simulink model "IEEE123_4subsystem"  (R2022b)
settings: Solver=ode4  StartTime=0.0  StopTime=inf  FixedStep=Ts  MaxStep=1e-4  RelTol=1e-3
PreLoadFcn:
  | Ts = 50e-6;
PostLoadFcn:
  | Ts = 50e-6;
InitFcn:
  | %%%%%%%%%%%%%%%%%%%%%%%%
  | % Simulation data for the IEEE 123 Node Test Feeder model
  | %%%%%%%%%%%%%%%%%%%%%%%
  | 
  | % miles/km
  | mi2km = 1.60934;
  | 
  | % feet to km
  | ft2km = 0.0003048;
  | 
  | % microsiemens to Farads
  | ms2F = 1/2/pi/60*1e-6;
  | 
  | %% Configuration 1 - series reactance - ohm/mile
  | 
  | R_1 = [0.4576 0.1560 0.1535;0.1560 0.4666 0.1580;0.1535 0.1580 0.4615];
  | X_1 = [1.0780 0.5017 0.3849;0.5017 1.0482 0.4236;0.3849 0.4236 1.0651];
  | 
  | % charging susceptance - microsiemens/mile
  | 
  | B_1 = [5.6765 -1.8319 -0.6982;-1.8319 5.9809 -1.1645;-0.6982 -1.1645 5.3971];
  | 
  | % convert for SPS
  | 
  | R_1 = R_1/mi2km;
  | 
  | Rs_1=(R_1(1,1)+R_1(2,2)+R_1(3,3))/3;
  | Rm_1=(R_1(1,2)+R_1(1,3)+R_1(2,3))/3;
  | R1_1=Rs_1-Rm_1;
  | R0_1=Rs_1+2*Rm_1;
  | 
  | L_1 = X_1/mi2km/2/pi/60;
  | 
  | Ls_1=(L_1(1,1)+L_1(2,2)+L_1(3,3))/3;
  | Lm_1=(L_1(1,2)+L_1(1,3)+L_1(2,3))/3;
  | L1_1=Ls_1-Lm_1;
  | L0_1=Ls_1+2*Lm_1;
  | 
  | C_1 = B_1/mi2km*ms2F;
  | 
  | Cs_1=(C_1(1,1)+C_1(2,2)+C_1(3,3))/3;
  | Cm_1=(C_1(1,2)+C_1(1,3)+C_1(2,3))/3;
  | C1_1=Cs_1-Cm_1;
  | C0_1=Cs_1+2*Cm_1;
  | 
  | 
  | %% Configuration 2 - series reactance - ohm/mile
  | 
  | R_2 = [0.4666 0.1580 0.1560;0.1580 0.4615 0.1535;0.1560 0.1535 0.4576];
  | X_2 = [1.0482 0.4236 0.5017;0.4236 1.0651 0.3849;0.5017 0.3849 1.0780];
  | 
  | % charging susceptance - microsiemens/mile
  | 
  | B_2 = [5.9809 -1.1645 -1.8319;-1.1645 5.3971 -0.6982;-1.8319 -0.6982 5.6765];
  | 
  | % convert for SPS
  | 
  | R_2 = R_2/mi2km;
  | 
  | Rs_2=(R_2(1,1)+R_2(2,2)+R_2(3,3))/3;
  | Rm_2=(R_2(1,2)+R_2(1,3)+R_2(2,3))/3;
  | R1_2=Rs_2-Rm_2;
  | R0_2=Rs_2+2*Rm_2;
  | 
  | L_2 = X_2/mi2km/2/pi/60;
  | 
  | Ls_2=(L_2(1,1)+L_2(2,2)+L_2(3,3))/3;
  | Lm_2=(L_2(1,2)+L_2(1,3)+L_2(2,3))/3;
  | L1_2=Ls_2-Lm_2;
  | L0_2=Ls_2+2*Lm_2;
  | 
  | C_2 = B_2/mi2km*ms2F;
  | 
  | Cs_2=(C_2(1,1)+C_2(2,2)+C_2(3,3))/3;
  | Cm_2=(C_2(1,2)+C_2(1,3)+C_2(2,3))/3;
  | C1_2=Cs_2-Cm_2;
  | C0_2=Cs_2+2*Cm_2;
  | 
  | 
  | %% Configuration 3 - series reactance - ohm/mile
  | 
  | R_3 = [0.4615 0.1535 0.1580;0.1535 0.4576 0.1560;0.1580 0.1560 0.4666];
  | X_3 = [1.0651 0.3849 0.4236;0.3849 1.0780 0.5017;0.4236 0.5017 1.0482];
  | 
  | % charging susceptance - microsiemens/mile
  | 
  | B_3 = [5.3971 -0.6982 -1.1645;-0.6982 5.6765 -1.8319; -1.1645 -1.8319 5.9809];
  | 
  | % convert for SPS
  | 
  | R_3 = R_3/mi2km;
  | 
  | Rs_3=(R_3(1,1)+R_3(2,2)+R_3(3,3))/3;
  | Rm_3=(R_3(1,2)+R_3(1,3)+R_3(2,3))/3;
  | R1_3=Rs_3-Rm_3;
  | R0_3=Rs_3+2*Rm_3;
  | 
  | L_3 = X_3/mi2km/2/pi/60;
  | 
  | Ls_3=(L_3(1,1)+L_3(2,2)+L_3(3,3))/3;
  | Lm_3=(L_3(1,2)+L_3(1,3)+L_3(2,3))/3;
  | L1_3=Ls_3-Lm_3;
  | L0_3=Ls_3+2*Lm_3;
  | 
  | C_3 = B_3/mi2km*ms2F;
  | 
  | Cs_3=(C_3(1,1)+C_3(2,2)+C_3(3,3))/3;
  | Cm_3=(C_3(1,2)+C_3(1,3)+C_3(2,3))/3;
  | C1_3=Cs_3-Cm_3;
  | C0_3=Cs_3+2*Cm_3;
  | 
  | %% Configuration 4 - series reactance - ohm/mile
  | 
  | R_4 = [0.4615 0.1580 0.1535;0.1580 0.4666 0.1560;0.1535 0.1560 0.4576];
  | X_4 = [1.0651 0.4236 0.3849;0.4236 1.0482 0.5017;0.3849 0.5017 1.0780];
  | 
  | % charging susceptance - microsiemens/mile
  | 
  | B_4 = [5.3971 -1.1645 -0.6982;-1.1645 5.9809 -1.8319;-0.6982 -1.8319 5.6765];
  | 
  | % convert for SPS
  | 
  | R_4 = R_4/mi2km;
  | 
  | Rs_4=(R_4(1,1)+R_4(2,2)+R_4(3,3))/3;
  | Rm_4=(R_4(1,2)+R_4(1,3)+R_4(2,3))/3;
  | R1_4=Rs_4-Rm_4;
  | R0_4=Rs_4+2*Rm_4;
  | 
  | L_4 = X_4/mi2km/2/pi/60;
  | 
  | Ls_4=(L_4(1,1)+L_4(2,2)+L_4(3,3))/3;
  | Lm_4=(L_4(1,2)+L_4(1,3)+L_4(2,3))/3;
  | L1_4=Ls_4-Lm_4;
  | L0_4=Ls_4+2*Lm_4;
  | 
  | C_4 = B_4/mi2km*ms2F;
  | 
  | Cs_4=(C_4(1,1)+C_4(2,2)+C_4(3,3))/3;
  | Cm_4=(C_4(1,2)+C_4(1,3)+C_4(2,3))/3;
  | C1_4=Cs_4-Cm_4;
  | C0_4=Cs_4+2*Cm_4;
  | 
  | 
  | %% Configuration 5 - series reactance - ohm/mile
  | 
  | R_5 = [0.4666 0.1560 0.1580;0.1560 0.4576 0.1535;0.1580 0.1535 0.4615];
  | X_5 = [1.0482 0.5017 0.4236;0.5017 1.0780 0.3849;0.4236 0.3849 1.0651];
  | 
  | % charging susceptance - microsiemens/mile
  | 
  | B_5 = [5.9809 -1.8319 -1.1645;-1.8319 5.6765 -0.6982;-1.1645 -0.6982 5.3971];
  | 
  | % convert for SPS
  | 
  | R_5 = R_5/mi2km;
  | 
  | Rs_5=(R_5(1,1)+R_5(2,2)+R_5(3,3))/3;
  | Rm_5=(R_5(1,2)+R_5(1,3)+R_5(2,3))/3;
  | R1_5=Rs_5-Rm_5;
  | R0_5=Rs_5+2*Rm_5;
  | 
  | L_5 = X_5/mi2km/2/pi/60;
  | 
  | Ls_5=(L_5(1,1)+L_5(2,2)+L_5(3,3))/3;
  | Lm_5=(L_5(1,2)+L_5(1,3)+L_5(2,3))/3;
  | L1_5=Ls_5-Lm_5;
  | L0_5=Ls_5+2*Lm_5;
  | 
  | C_5 = B_5/mi2km*ms2F;
  | 
  | Cs_5=(C_5(1,1)+C_5(2,2)+C_5(3,3))/3;
  | Cm_5=(C_5(1,2)+C_5(1,3)+C_5(2,3))/3;
  | C1_5=Cs_5-Cm_5;
  | C0_5=Cs_5+2*Cm_5;
  | 
  | %% Configuration 6 - series reactance - ohm/mile
  | 
  | R_6 = [0.4576 0.1535 0.1560;0.1535 0.4615 0.1580;0.1560 0.1580 0.4666];
  | X_6 = [1.0780 0.3849 0.5017;0.3849 1.0651 0.4236;0.5017 0.4236 1.0482];
  | 
  | % charging susceptance - microsiemens/mile
  | 
  | B_6 = [5.6765 -0.6982 -1.8319;-0.6982 5.3971 -1.1645;-1.8319 -1.1645 5.9809];
  | 
  | % convert for SPS
  | 
  | R_6 = R_6/mi2km;
  | 
  | Rs_6=(R_6(1,1)+R_6(2,2)+R_6(3,3))/3;
  | Rm_6=(R_6(1,2)+R_6(1,3)+R_6(2,3))/3;
  | R1_6=Rs_6-Rm_6;
  | R0_6=Rs_6+2*Rm_6;
  | 
  | L_6 = X_6/mi2km/2/pi/60;
  | 
  | Ls_6=(L_6(1,1)+L_6(2,2)+L_6(3,3))/3;
  | Lm_6=(L_6(1,2)+L_6(1,3)+L_6(2,3))/3;
  | L1_6=Ls_6-Lm_6;
  | L0_6=Ls_6+2*Lm_6;
  | 
  | C_6 = B_6/mi2km*ms2F;
  | 
  | Cs_6=(C_6(1,1)+C_6(2,2)+C_6(3,3))/3;
  | Cm_6=(C_6(1,2)+C_6(1,3)+C_6(2,3))/3;
  | C1_6=Cs_6-Cm_6;
  | C0_6=Cs_6+2*Cm_6;
  | 
  | 
  | %% Configuration 7 - series reactance - ohm/mile
  | 
  | R_7 = [0.4576 0.0000 0.1535;0.0000 0.0000 0.0000;0.1535 0.0000 0.4615];
  | X_7 = [1.0780 0.0000 0.3849;0.0000 0.0000 0.0000;0.3849 0.0000 1.0651];
  | 
  | % charging susceptance - microsiemens/mile
  | 
  | B_7 = [5.1154 0.0000 -1.0549;0.0000 0.0000 0.0000;-1.0549 0.0000 5.1704];
  | 
  | % convert for SPS
  | 
  | R_7 = R_7/mi2km;
  | 
  | Rs_7=(R_7(1,1)+R_7(2,2)+R_7(3,3))/3;
  | Rm_7=(R_7(1,2)+R_7(1,3)+R_7(2,3))/3;
  | R1_7=Rs_7-Rm_7;
  | R0_7=Rs_7+2*Rm_7;
  | 
  | L_7 = X_7/mi2km/2/pi/60;
  | 
  | Ls_7=(L_7(1,1)+L_7(2,2)+L_7(3,3))/3;
  | Lm_7=(L_7(1,2)+L_7(1,3)+L_7(2,3))/3;
  | L1_7=Ls_7-Lm_7;
  | L0_7=Ls_7+2*Lm_7;
  | 
  | C_7 = B_7/mi2km*ms2F;
  | 
  | Cs_7=(C_7(1,1)+C_7(2,2)+C_7(3,3))/3;
  | Cm_7=(C_7(1,2)+C_7(1,3)+C_7(2,3))/3;
  | C1_7=Cs_7-Cm_7;
  | C0_7=Cs_7+2*Cm_7;
  | 
  | 
  | %% Configuration 8 - series reactance - ohm/mile
  | 
  | R_8 = [0.4576 0.1535 0.0000;0.1535 0.4615 0.0000;0.0000 0.0000 0.0000];
  | X_8 = [1.0780 0.3849 0.0000;0.3849 1.0651 0.0000;0.0000 0.0000 0.0000];
  | 
  | % charging susceptance - microsiemens/mile
  | 
  | B_8 = [5.1154 -1.0549 0.0000;-1.0549 5.1704 0.0000;0.0000 0.0000 0.0000];
  | 
  | % convert for SPS
  | 
  | R_8 = R_8/mi2km;
  | 
  | Rs_8=(R_8(1,1)+R_8(2,2)+R_8(3,3))/3;
  | Rm_8=(R_8(1,2)+R_8(1,3)+R_8(2,3))/3;
  | R1_8=Rs_8-Rm_8;
  | R0_8=Rs_8+2*Rm_8;
  | 
  | L_8 = X_8/mi2km/2/pi/60;
  | 
  | Ls_8=(L_8(1,1)+L_8(2,2)+L_8(3,3))/3;
  | Lm_8=(L_8(1,2)+L_8(1,3)+L_8(2,3))/3;
  | L1_8=Ls_8-Lm_8;
  | L0_8=Ls_8+2*Lm_8;
  | 
  | C_8 = B_8/mi2km*ms2F;
  | 
  | Cs_8=(C_8(1,1)+C_8(2,2)+C_8(3,3))/3;
  | Cm_8=(C_8(1,2)+C_8(1,3)+C_8(2,3))/3;
  | C1_8=Cs_8-Cm_8;
  | C0_8=Cs_8+2*Cm_8;
  | 
  | %% Configuration 9 - series reactance - ohm/mile
  | 
  | R_9 = [1.3292 0 0;0 0 0;0 0 0];
  | X_9 = [1.3475 0 0;0 0 0;0 0 0];
  | 
  | % charging susceptance - microsiemens/mile
  | 
  | B_9 = [4.5193 0 0;0 0 0;0 0 0];
  | 
  | % convert for SPS
  | 
  | R_9 = R_9/mi2km;
  | 
  | Rs_9=(R_9(1,1)+R_9(2,2)+R_9(3,3))/3;
  | Rm_9=(R_9(1,2)+R_9(1,3)+R_9(2,3))/3;
  | R1_9=Rs_9-Rm_9;
  | R0_9=Rs_9+2*Rm_9;
  | 
  | L_9 = X_9/mi2km/2/pi/60;
  | 
  | Ls_9=(L_9(1,1)+L_9(2,2)+L_9(3,3))/3;
  | Lm_9=(L_9(1,2)+L_9(1,3)+L_9(2,3))/3;
  | L1_9=Ls_9-Lm_9;
  | L0_9=Ls_9+2*Lm_9;
  | 
  | C_9 = B_9/mi2km*ms2F;
  | 
  | Cs_9=(C_9(1,1)+C_9(2,2)+C_9(3,3))/3;
  | Cm_9=(C_9(1,2)+C_9(1,3)+C_9(2,3))/3;
  | C1_9=Cs_9-Cm_9;
  | C0_9=Cs_9+2*Cm_9;
  | 
  | %% Configuration 10- series reactance - ohm/mile
  | 
  | R_10 = [0 0 0;0 1.3292 0;0 0 0];
  | X_10 = [0 0 0;0 1.3475 0;0 0 0];
  | 
  | % charging susceptance - microsiemens/mile
  | B_10 = [0 0 0;0 4.5193 0;0 0 0];
  | 
  | % convert for SPS
  | 
  | R_10 = R_10/mi2km;
  | 
  | Rs_10=(R_10(1,1)+R_10(2,2)+R_10(3,3))/3;
  | Rm_10=(R_10(1,2)+R_10(1,3)+R_10(2,3))/3;
  | R1_10=Rs_10-Rm_10;
  | R0_10=Rs_10+2*Rm_10;
  | 
  | L_10 = X_10/mi2km/2/pi/60;
  | 
  | Ls_10=(L_10(1,1)+L_10(2,2)+L_10(3,3))/3;
  | Lm_10=(L_10(1,2)+L_10(1,3)+L_10(2,3))/3;
  | L1_10=Ls_10-Lm_10;
  | L0_10=Ls_10+2*Lm_10;
  | 
  | C_10 = B_10/mi2km*ms2F;
  | 
  | Cs_10=(C_10(1,1)+C_10(2,2)+C_10(3,3))/3;
  | Cm_10=(C_10(1,2)+C_10(1,3)+C_10(2,3))/3;
  | C1_10=Cs_10-Cm_10;
  | C0_10=Cs_10+2*Cm_10;
  | 
  | %% Configuration 11 - series reactance - ohm/mile
  | 
  | R_11 = [0 0 0;0 0 0;0 0 1.3292];
  | X_11 = [0 0 0;0 0 0;0 0 1.3475];
  | 
  | % charging susceptance - microsiemens/mile
  | 
  | B_11 = [0 0 0;0 0 0;0 0 4.5193];
  | 
  | % convert for SPS
  | 
  | R_11 = R_11/mi2km;
  | 
  | Rs_11=(R_11(1,1)+R_11(2,2)+R_11(3,3))/3;
  | Rm_11=(R_11(1,2)+R_11(1,3)+R_11(2,3))/3;
  | R1_11=Rs_11-Rm_11;
  | R0_11=Rs_11+2*Rm_11;
  | 
  | L_11 = X_11/mi2km/2/pi/60;
  | 
  | Ls_11=(L_11(1,1)+L_11(2,2)+L_11(3,3))/3;
  | Lm_11=(L_11(1,2)+L_11(1,3)+L_11(2,3))/3;
  | L1_11=Ls_11-Lm_11;
  | L0_11=Ls_11+2*Lm_11;
  | 
  | C_11 = B_11/mi2km*ms2F;
  | 
  | Cs_11=(C_11(1,1)+C_11(2,2)+C_11(3,3))/3;
  | Cm_11=(C_11(1,2)+C_11(1,3)+C_11(2,3))/3;
  | C1_11=Cs_11-Cm_11;
  | C0_11=Cs_11+2*Cm_11;
  | 
  | 
  | %% Configuration 12 - series reactance - ohm/mile
  | 
  | R_12 = [1.5209 0.5198 0.4924;0.5198 1.5329 0.5198;0.4924 0.5198 1.5209];
  | X_12 = [0.7521 0.2775 0.2157;0.2775 0.7162 0.2775;0.2157 0.2775 0.7521];
  | 
  | % charging susceptance - microsiemens/mile
  | 
  | B_12 = [67.2242 0.0000 0.0000;0.0000 67.2242 0.0000;0.0000 0.0000 67.2242];
  | 
  | % convert for SPS
  | 
  | R_12 = R_12/mi2km;
  | 
  | Rs_12=(R_12(1,1)+R_12(2,2)+R_12(3,3))/3;
  | Rm_12=(R_12(1,2)+R_12(1,3)+R_12(2,3))/3;
  | R1_12=Rs_12-Rm_12;
  | R0_12=Rs_12+2*Rm_12;
  | 
  | L_12 = X_12/mi2km/2/pi/60;
  | 
  | Ls_12=(L_12(1,1)+L_12(2,2)+L_12(3,3))/3;
  | Lm_12=(L_12(1,2)+L_12(1,3)+L_12(2,3))/3;
  | L1_12=Ls_12-Lm_12;
  | L0_12=Ls_12+2*Lm_12;
  | 
  | C_12 = B_12/mi2km*ms2F;
  | 
  | Cs_12=(C_12(1,1)+C_12(2,2)+C_12(3,3))/3;
  | Cm_12=(C_12(1,2)+C_12(1,3)+C_12(2,3))/3;
  | C1_12=Cs_12-Cm_12;
  | C0_12=Cs_12+2*Cm_12;
undefined symbols (not defined in the file): D1, Delta, find_system, I, Left, MOV_segment9, powergui, Right, type, V, X
libraries: spsGroundLib x242, spsThreePhaseVIMeasurementLib x134, spsSeriesRLCBranchLib x107, spsSeriesRLCLoadLib x83, spsPiSectionLineLib x61, spsThreePhasePISectionLineLib x60, spsVoltageMeasurementLib x52, spsDCVoltageSourceLib x36, ssn_lib x28, artemis x24, spsACCurrentSourceLib x18, spsOnDelayLib x18
(part 1 of 15)
settings Model: ARTEMISmethode_block_infos=$$__separator__$$IEEE123_4subsystem/ARTEMIS Guide$$__separator__$$  Creator=Arun  LastModifiedBy=AS7434
settings SolverCC: AlgebraicLoopSolver=TrustRegion
settings DataIOCC: ReturnWorkspaceOutputs=off
settings DebuggingCC: SFMachineParentedDataDiag=warning  ArithmeticOperatorsInVariantConditions=warning
settings ModelReferenceCC: EnableRefExpFcnMdlSchedulingChecks=on
settings SFSimCC: SimUseLocalCustomCode=off  CustomCodeUndefinedFunction=UseInterfaceOnly
settings RTWCC: RTWUseLocalCustomCode=off
settings CodeAppCC: StateflowObjectComments=on
settings SimscapeCC: SimscapeNormalizeSystem=off

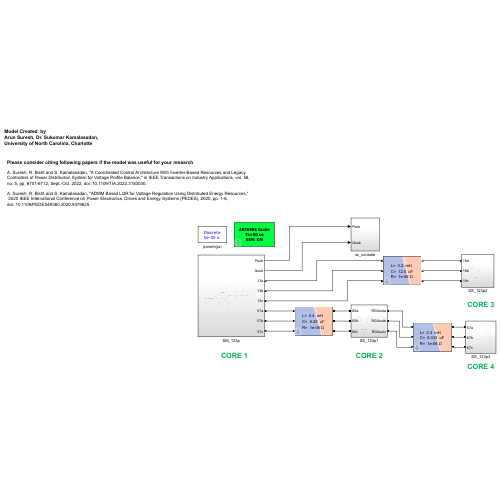
[thumbnail: Simulink's stored preview of the top-level diagram]
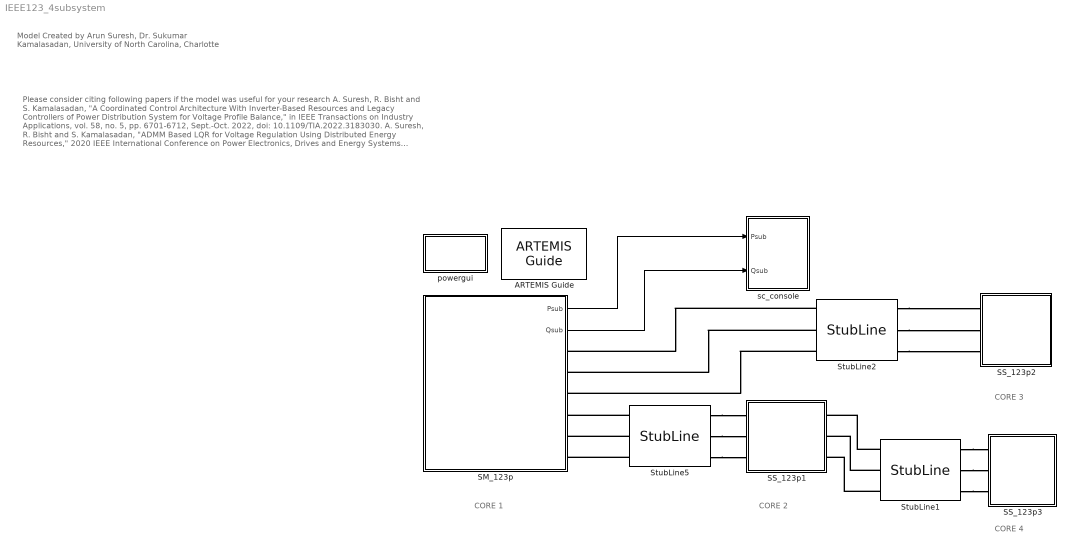
== system IEEE123_4subsystem ==
  note: CORE 1
  note: CORE 2
  note: CORE 3
  note: CORE 4
  note: Model Created by
      | Arun Suresh, Dr. Sukumar Kamalasadan,
      | University of North Carolina, Charlotte
  note: Please consider citing following papers if the model was useful for your research
      |
      | A. Suresh, R. Bisht and S. Kamalasadan, "A Coordinated Control Architecture With Inverter-Based Resources and Legacy
      | Controllers of Power Distribution System for Voltage Profile Balance," in IEEE Transactions on Industry Applications, vol. 58,
      | no. 5, pp. 6701-6712, Sept.-Oct. 2022, doi: 10.1109/TIA.2022.3183030.
      |
      | A. Suresh, R. Bisht and S. Kamalasadan, "ADMM Based LQR for Voltage Regulation Using Distributed Energy Resources,"
      | 2020 IEEE International Conference on Power Electronics, Drives and Energy Systems (PEDES), 2020, pp. 1-6,
      | doi: 10.1109/PEDES49360.2020.9379625.
  ARTEMIS Guide : artemis/ARTEMIS/ARTEMIS Guide  Tag=FTSSmethode_opal_4hx0r99  Description=5.0_z1  lock=on  Ts=Ts  ssn=on  opt=art5  dyna=off  nb_perm=4  RT_fullcomp=off  ssn_itvc=off  ssn_ivic=off  ssn_ext=off  ssn_solver=Art5  iter_type=iSWITCH and iMOV only (default)  ssn_ImpulseLoopBlockedStateUpdate=2  ssn_mov_iter_number=2  ssn_switch_iter_number=2  ssn_lu_or_ldlt=LU (more robust)  ssn_nib_type_verify=off  ssn_use_lu=on  ssn_use_ldlt=off  ssn_impulse=on  ssn_quasimpulse=off  ssn_impulse_loop=2  paraExtinctionThy=off  Thy_Impulse=on  dtc=Off  dtc_opt=normal  ao=on  simtype=off  ct_mac=off  lin_mov=off  lsp=[0.001 2]  spike_skip=Disabled  dtc_extra=1  dtc_sws=normal  dtc_pied=0.5  SPSRulesBlock=SPSRules  tre=on  ctmm=off  LF=off  dpl_type=ARTEMiS DPL  rlc_type=off  custom_type=off  para=on  ssn_full_iteration=off  ssn_init_cond=block only
  SM_123p : Subsystem
  SS_123p1 : Subsystem
  SS_123p2 : Subsystem
  SS_123p3 : Subsystem
  StubLine1 : artemis/ARTEMIS/StubLine  Phases=3  pu=off  L=3e-4  Lpu=0.004  R=1e-6  Rpu=0.001  S_base=5e6  V_base=4160  F_base=60  Ts=Ts
  StubLine2 : artemis/ARTEMIS/StubLine  Phases=3  pu=off  L=2e-4  Lpu=0.004  R=1e-6  Rpu=0.001  S_base=5e6  V_base=4160  F_base=60  Ts=Ts
  StubLine5 : artemis/ARTEMIS/StubLine  Phases=3  pu=off  L=4e-4  Lpu=0.004  R=1e-6  Rpu=0.001  S_base=5e6  V_base=4160  F_base=60  Ts=Ts
  powergui : Subsystem  Priority=1  DialogController=POWERSYS.PowerSysDialog  InitFcn=powergui( 'InitFcn_Callback' , gcb , 0 , [ ] );  mask(PSB option menu block){SimulationMode=Discrete, SampleTime=Ts, frequency=60, Iterations=50, frequencyindice=0, Pbase=100e6, ErrMax=1e-4, UnitsV=kV, UnitsW=MW, buscounter=0, FunctionMessages=off, echomessages=on, EnableUseOfTLC=off, CurrentSourceSwitches=off, DisableSnubberDevices=off, DisableRonSwitches=off, DisableVfSwitches=off, DisplayEquations=off, AutomaticDiscreteSolvers=off, SolverType=Tustin/Backward Euler (TBE), Interpol=off, ExternalGateDelay=off, methode=off, Ts=0, x0status=blocks, SPID=off, SwTol=0, HookPort=off, NonlinearTolerance=1e-4, nMaxIteration=100, ContinueOnMaxIteration=off, RestoreLinks=warning, ResistiveCurrentMeasurement=off, Frange=[0:2:500], Ylog=off, Xlog=on, ShowGrid=off, save=off, variable=ZData, structure=0, ZoomFFT=off, StartTime=0.0, cycles=1, DisplayStyle=1, fundamental=60, FreqAxis=off, MaxFrequency=1000, frequencyindicesteady=1, RmsSteady=1, display=off}
      mask prompts: SimulationMode "Simulation type:"; SampleTime "Sample time (s):"; frequency "Frequency (Hz):"; Iterations "Max iterations"; frequencyindice "Frequency (Hz)"; Pbase "Base power (VA)"; ErrMax "PQ tolerance (pu)"; UnitsV "Voltage units"; UnitsW "Power units"; buscounter "Load flow bus counter"; FunctionMessages "Disable Specialized Power Systems warnings"; echomessages "Display Specialized Power Systems compilation messages"; EnableUseOfTLC "Use TLC file when in Accelerator Simulation Mode and for code generation"; CurrentSourceSwitches "Disable ideal switching"; DisableSnubberDevices "Disable snubbers in switching devices"; DisableRonSwitches "Disable Ron resistances in switching devices"; DisableVfSwitches "Disable forward voltages in switching devices"; DisplayEquations "Display circuit differential equations"; AutomaticDiscreteSolvers "Automatically handle Discrete solver and Advanced tab solver settings of blocks"; SolverType "Discrete solver"; Interpol "Interpolate switching events"; ExternalGateDelay "Use time-stamped gate signals"; methode "Store switching topologies"; Ts "Buffer size (MBytes):"; x0status "Start simulation with initial electrical states from:"; SPID "Use ideal switching devices"; SwTol "Switch tolerance"; HookPort "Allow multiple powergui blocks"; NonlinearTolerance "Solver tolerance"; nMaxIteration "Maximum number of iterations"; ContinueOnMaxIteration "Continue Simulation if maximum number of iterations is reached"; RestoreLinks "Restore disabled links of Simscape Power Systems ST blocks:"; ResistiveCurrentMeasurement "Use non ideal current measurement blocks (1e-4Ohm internal resistance)"; Frange "Frequency Range"; Ylog "Log impedance"; Xlog "log Frequency"; ShowGrid "grid"; save "Save Data To Workspace"; variable "Variable Name"; structure "Structure Name (PSBFFTSCOPE)"; ZoomFFT "ZoomFFT (PSBFFTSCOPE)"; StartTime "Start Time (PSBFFTSCOPE)"; cycles "Cycles (PSBFFTSCOPE)"; DisplayStyle "Display style (PSBFFTSCOPE)"; fundamental "Fundamental (PSBFFTSCOPE)"; FreqAxis "Frequency Axis (PSBFFTSCOPE)"; MaxFrequency "Max Frequency (PSBFFTSCOPE)"; frequencyindicesteady "Frequency indice (STEADYSTATE)"; RmsSteady "RMS display (STEADYSTATE)"; display "Display Results"
      mask help: Set simulation type, simulation parameters, and preferences.
      mask init:
      | dispMessage = powergui('MaskInitialization',gcb,SimulationMode,SampleTime);
      settings: LibrarySourceBlock=sps_lib/powergui  PreSaveFcn=powergui( 'PreSaveFcn_Callback' , gcb , [ ] , [ ] );  OpenFcn=sps_rtmsupport('OpenFcn',gcbh)
      mask Help: helpview(psbhelp)
      mask TypeOptions SimulationMode: Continuous | Discrete | Phasor | Discrete phasor
      mask Callback SimulationMode: powergui('SimulationType',[],[],gcb);
      mask TypeOptions UnitsV: V | kV
      mask TypeOptions UnitsW: W | kW | MW
      mask Callback CurrentSourceSwitches: powergui('SimulationType',[],[],gcb);
      mask Callback AutomaticDiscreteSolvers: powergui('SimulationType',[],[],gcb);
      mask TypeOptions SolverType: Tustin/Backward Euler (TBE) | Tustin | Backward Euler
      mask Callback SolverType: powergui('SimulationType',[],[],gcb);
      mask Callback Interpol: powergui('SimulationType',[],[],gcb);
      mask Callback ExternalGateDelay: powergui('SimulationType',[],[],gcb);
      mask Callback methode: powergui('SimulationType',[],[],gcb);
      mask TypeOptions x0status: blocks | steady | zero
      mask TypeOptions RestoreLinks: yes | warning | no
      mask Callback display: sps_rtmsupport('parametereditingmodes',gcbh) % Will be executed last in parameter callbacks to ensure mask enable consistency
      mask DialogControl SolverTab Prompt: Solver
      mask DialogControl AutoSolverNote Prompt: The Simulation type parameter is governed by Simulink. To access the Powergui solver settings, unselect auto (Automatic solver selection) solver in the Simulink solver options.
      mask DialogControl Container15 Prompt: Tools
      mask DialogControl StateAnalyzer Prompt: Measurements and States Analyzer
      mask DialogControl StateAnalyzer Callback: powerStates(bdroot(gcb))
      mask DialogControl RLCLineParameters Prompt: Power Line Parameters
      mask DialogControl RLCLineParameters Callback:
      | close_system(gcb)
      | powerLineParameters
      mask DialogControl Control15 Prompt: Power Cable Parameters
      mask DialogControl Control15 Callback:
      | close_system(gcb)
      | powerCableParameters
      mask DialogControl DecouplingLines Prompt: Specify Decoupling Lines
      mask DialogControl DecouplingLines Tooltip: Click to replace selected Distributed Parameters Line blocks with Decoupling Line blocks
      mask DialogControl DecouplingLines Callback:
      | close_system(gcb);
      | DecouplingLineReplace(gcs)
      mask DialogControl LoadFlow Prompt: Load Flow Analyzer
      mask DialogControl LoadFlow Callback:
      | close_system(gcb)
      | powerLoadFlow
      mask DialogControl Container11 Prompt: Load Flow Parameters
      mask DialogControl MachineInitialization Prompt: Machine Initialization
      mask DialogControl MachineInitialization Callback:
      | close_system(gcb)
      | powericon('machineInitTool',bdroot(gcb),gcb)
      mask DialogControl ImpedanceMeasurement Prompt: Impedance Measurement
      mask DialogControl ImpedanceMeasurement Callback:
      | close_system(gcb);
      | powerImpedance(bdroot(gcs));
      mask DialogControl FFTAnalysis Prompt: FFT Analysis
      mask DialogControl FFTAnalysis Callback:
      | close_system(gcb)
      | power_fftscope(bdroot(gcb),gcb)
      mask DialogControl LinearSystemAnalyzer Prompt: Use Linear System Analyzer
      mask DialogControl LinearSystemAnalyzer Callback:
      | close_system(gcb)
      | power_ltiview(bdroot(gcb))
      mask DialogControl HysteresisDesign Prompt: Hysteresis Design
      mask DialogControl HysteresisDesign Callback:
      | close_system(gcb)
      | powerHysteresis('hysteresis.mat')
      mask DialogControl Control14 Prompt: Customize SPS blocks
      mask DialogControl Control14 Callback:
      | close_system(gcb);
      | power_customize;
      mask DialogControl GenerateReprot Prompt: Generate Report
      mask DialogControl GenerateReprot Callback:
      | close_system(gcb)
      | power_report(bdroot(gcb))
      mask DialogControl ParameterTabVar012 Prompt: Preferences
      mask DialogControl Solver Prompt: Solver
      mask DialogControl SolverDetails Prompt: Solver details for nonlinear elements
      mask Display: color('blue'),disp(dispMessage)
  sc_console : Subsystem
  wires:
  SM_123p/2(Qsub) -> sc_console/2(Qsub)
  SM_123p/1(Psub) -> sc_console/1(Psub)
  connections:
  StubLine5/RConn1 -- SS_123p1/LConn1
  StubLine5/RConn2 -- SS_123p1/LConn2
  StubLine5/RConn3 -- SS_123p1/LConn3
  StubLine5/LConn3 -- SM_123p/RConn6
  StubLine5/LConn2 -- SM_123p/RConn5
  StubLine5/LConn1 -- SM_123p/RConn4
  StubLine1/LConn2 -- SS_123p1/RConn2
  StubLine1/LConn1 -- SS_123p1/RConn1
  StubLine1/LConn3 -- SS_123p1/RConn3
  StubLine1/RConn1 -- SS_123p3/LConn1
  StubLine1/RConn2 -- SS_123p3/LConn2
  StubLine1/RConn3 -- SS_123p3/LConn3
  StubLine2/RConn2 -- SS_123p2/LConn2
  StubLine2/RConn1 -- SS_123p2/LConn1
  StubLine2/RConn3 -- SS_123p2/LConn3
  StubLine2/LConn3 -- SM_123p/RConn3
  StubLine2/LConn2 -- SM_123p/RConn2
  StubLine2/LConn1 -- SM_123p/RConn1
